simulink model "family_1_variant_2_PlayBack_Data"  (R2014a)
settings: Solver=ode45  StartTime=0.0  StopTime=Recorded_Accelerometer.time(end)  FixedStep=1/400  RelTol=1e-3
undefined symbols (not defined in the file): Accelerometer_360deg_calibration
settings Model: Creator=darenlee  LastModifiedBy=Raphaël
settings OptimizationCC: SimCompilerOptimization=off
settings DebuggingCC: MergeDetectMultiDrivingBlocksExec=error  FrameProcessingCompatibilityMsg=error
settings RTWCC: RTWCompilerOptimization=off

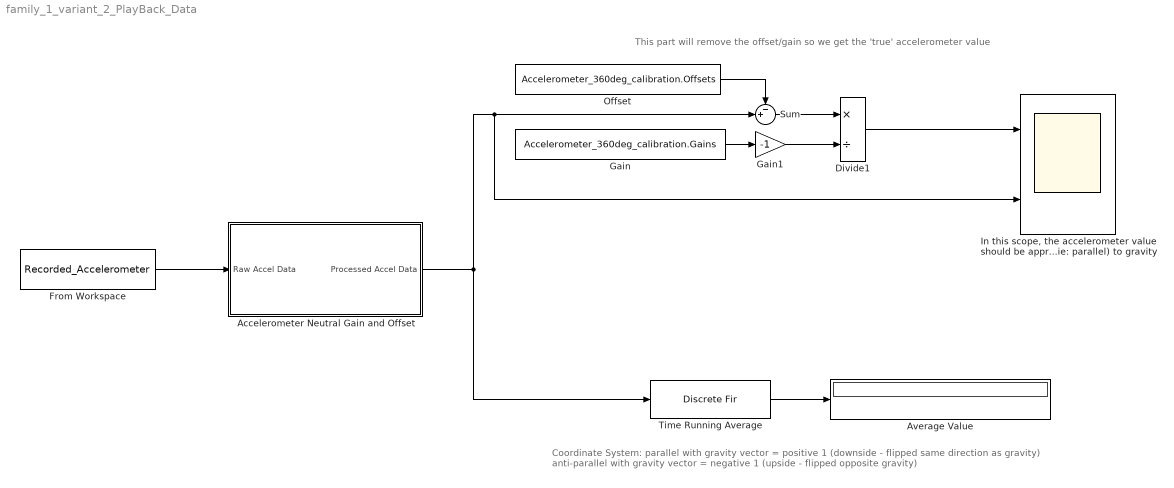
== system family_1_variant_2_PlayBack_Data ==
  note: Coordinate System: parallel with gravity vector = positive 1    (downside - flipped same direction as gravity)
      |                                 anti-parallel with gravity vector = negative 1   (upside - flipped opposite gravity)
  note: This part will remove the offset/gain so we get the 'true' accelerometer value
  Accelerometer Neutral Gain and Offset : Subsystem
  Average Value : Display
  Divide1 : Product  Inputs=*/
  From Workspace : FromWorkspace  VariableName=Recorded_Accelerometer  SampleTime=1/400
  Gain : Constant  Value=Accelerometer_360deg_calibration.Gains
  Gain1 : Gain  Gain=-1
  "In this scope, the accelerometer value should be approximately 1 for 1 axis and 0 for the other 2 axis. The data was recorded with each axis perfectly aligned (ie: parallel) to gravity" : Scope  NumInputPorts=2
      settings: TimeRange=7.423345884884347  YMin=-0.03831037494310437~0.4471153846153855  YMax=0.04794829597177959~1.249038461538462  SaveName=ScopeData2
  Offset : Constant  Value=Accelerometer_360deg_calibration.Offsets
  Sum : Sum  Inputs=-+|
  Time Running Average : DiscreteFir  Coefficients=ones(1,100)*(1/100)  SampleTime=1/400
  wires:
  From Workspace/1 -> Accelerometer Neutral Gain and Offset/1(Raw Accel Data)
  Time Running Average/1 -> Average Value/1
  Sum/1 -> Divide1/1
  Divide1/1 -> "In this scope, the accelerometer value should be approximately 1 for 1 axis and 0 for the other 2 axis. The data was recorded with each axis perfectly aligned (ie: parallel) to gravity"/1
  Gain/1 -> Gain1/1
  Gain1/1 -> Divide1/2
  Offset/1 -> Sum/1
  Accelerometer Neutral Gain and Offset/1(Processed Accel Data) -> Time Running Average/1, Sum/2, "In this scope, the accelerometer value should be approximately 1 for 1 axis and 0 for the other 2 axis. The data was recorded with each axis perfectly aligned (ie: parallel) to gravity"/2

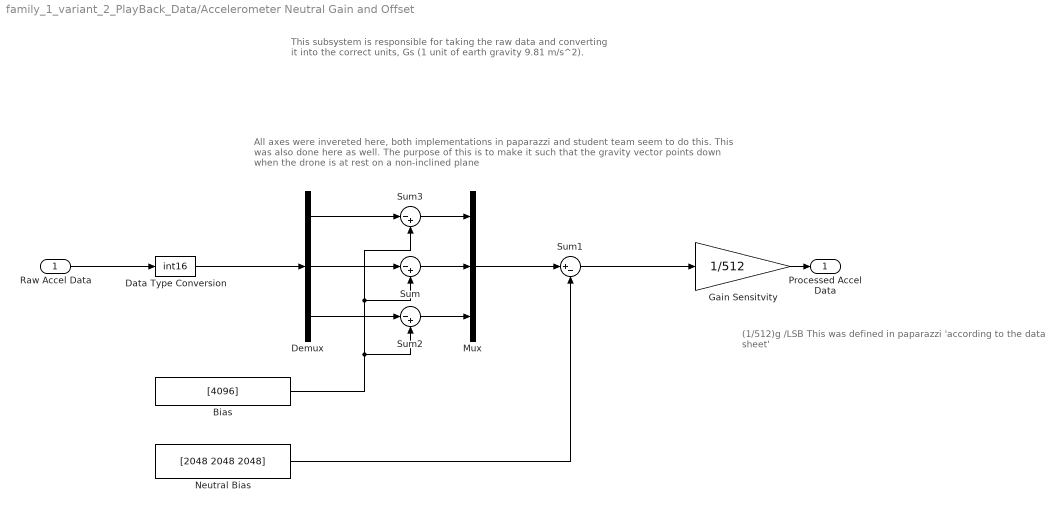
== system family_1_variant_2_PlayBack_Data/Accelerometer Neutral Gain and Offset ==
  note: This subsystem is responsible for taking the raw data and converting it into the correct units, Gs (1 unit of earth gravity 9.81 m/s^2).
  note: All axes were invereted here, both implementations in paparazzi and student
      |  team seem to do this. This was also done here as well. The purpose of this is to
      | make it such that the gravity vector points down when the drone is at rest on a non-inclined plane
  note: (1/512)g /LSB
      | This was defined in paparazzi 'according to the data sheet'
  Raw Accel Data : Inport
  Bias : Constant  Value=[4096]
  Data Type Conversion : DataTypeConversion  OutDataTypeStr=int16
  Demux : Demux  Outputs=3
  Gain Sensitvity : Gain  Gain=1/512
  Mux : Mux  Inputs=3
  Neutral Bias : Constant  Value=[2048 2048 2048]
  Sum : Sum  Inputs=|-+
  Sum1 : Sum  Inputs=|+-
  Sum2 : Sum  Inputs=|-+
  Sum3 : Sum  Inputs=|-+
  Processed Accel Data : Outport
  wires:
  Sum1/1 -> Gain Sensitvity/1
  Gain Sensitvity/1 -> Processed Accel Data/1
  Mux/1 -> Sum1/1
  Neutral Bias/1 -> Sum1/2
  Raw Accel Data/1 -> Data Type Conversion/1
  Sum3/1 -> Mux/1
  Demux/2 -> Sum/1
  Sum/1 -> Mux/2
  Demux/3 -> Sum2/1
  Sum2/1 -> Mux/3
  Bias/1 -> Sum2/2, Sum/2, Sum3/2
  Data Type Conversion/1 -> Demux/1
  Demux/1 -> Sum3/1
